simulink subsystem "ReqRestTimeCalc_Subsys"  (R2022b)
settings: Solver=VariableStepAuto  StartTime=0.0  StopTime=10.0  RelTol=1e-3
settings Model: Creator=Niharika  LastModifiedBy=Niharika

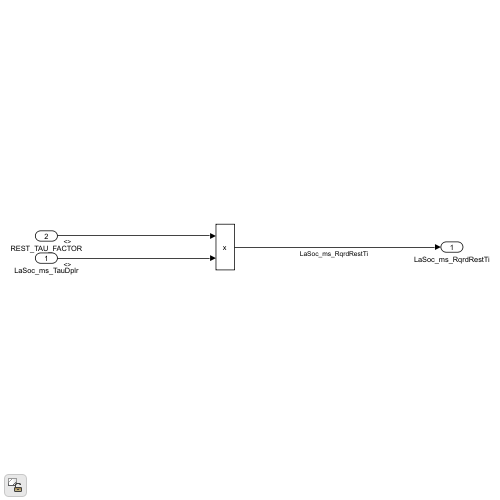
[thumbnail: Simulink's stored preview of the top-level diagram]
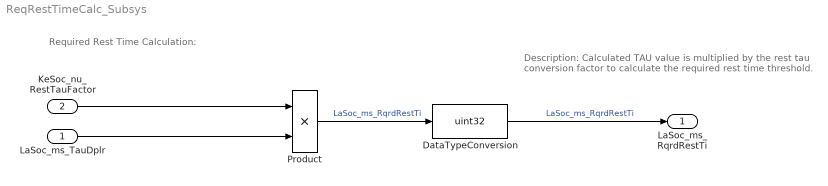
== system ReqRestTimeCalc_Subsys ==
  note: Description:
      | Calculated TAU value is multiplied by the rest tau conversion factor to calculate the required rest time threshold.
  note: Required Rest Time Calculation:
  LaSoc_ms_TauDplr : Inport
  KeSoc_nu_RestTauFactor : Inport  Port=2
  DataTypeConversion : DataTypeConversion  OutDataTypeStr=uint32  SaturateOnIntegerOverflow=off  RndMeth=Floor
  Product : Product
  LaSoc_ms_RqrdRestTi : Outport
  wires:
  Product/1 -> DataTypeConversion/1  "LaSoc_ms_RqrdRestTi"
  LaSoc_ms_TauDplr/1 -> Product/2
  KeSoc_nu_RestTauFactor/1 -> Product/1
  DataTypeConversion/1 -> LaSoc_ms_RqrdRestTi/1  "LaSoc_ms_RqrdRestTi"
